simulink model "ZEH_PV_grid"  (R2020a)
settings: Solver=VariableStepAuto  StartTime=0.0  StopTime=24*60*60  RelTol=1e-3
InitFcn:
  | SENSE2_dat
values from neighbouring files (symbols this model uses):
  apv = [72 76 288 252 0 0 40 360 460 168 84]  *1E2    [ZEH_dat_summer.m]    (also in ZEH_dat_winter.m)
  cab = [0.206 0.29 0.36 285 335 ... (first row only)    [ZEH_dat_summer.m]    (also in ZEH_dat_winter.m)
  cons = [0.64,0.60,0.58,0.56,0.56,0.58,0.64,0.76,0.87,0.95,0.99,1.00,0.99,1.00,1.00,0.97,0.96,0.96,0.93,0.92,0.92,0.93,0.87,0.72]    [ZEH_dat_summer.m]    (also in ZEH_dat_winter.m = [0.67,0.63,0.60,0.59,0.59,0.60,0.74,0.86,0.85,0.96,0.96,0.95)
  inic = 0.00095    [ZEH_dat_summer.m]    (also in ZEH_dat_winter.m)
  irr = [0,0,0,0,0,0,0,0,0,0,0,0,0,0,0,0,0,0,0,0,0,0,0,0,0,0,0,0,0,0,0,0,0,0,0,0,0,0,0,0,0,0,0,0,0,0,0,0,0,0,0,0,0,0,0,0,0,0,0,0,0,0,0,0,0,0,0,0,0,0,0,0,0,0,0,0,0,0,0,0,0,0,0,0,0,0,0,0,0,0,0,0,0,0,0,0,0,0,0,0,0,0,0,0,0,0,0,0,0,0,0,0,0,0,0,0,0,0,0,0,0,0,0,0,0,0,0,0,0,0,0,0,0,0,0,0,0,0,0,0,0,0,0,0,0,0,0,0,0,0,0,0,0,0,0,0,0,0,0,0,0,0,0,0,0,0,0,0,0,0,0,0,0,0,0,0,0,0,0,0,0,0,0,0,0,0,0,0,0,0,0,0,0,0,0,0,0,0,0,0 ...(+12851 chars)    [ZEH_dat_summer.m]    (also in ZEH_dat_winter.m = zeros(1,length(irr)))
  lp = 0.002    [ZEH_dat_summer.m]    (also in ZEH_dat_winter.m)
  SL = [7.57 8.06 30.73 53.01 133.26 219.22 4.00 37.53 48.38 17.80 9.04]*1E-3    [ZEH_dat_summer.m]    (also in ZEH_dat_winter.m)
  time = [1,1.01666666666667,1.03333333333333,1.05000000000000,1.06666666666667,1.08333333333333,1.10000000000000,1.11666666666667,1.13333333333333,1.15000000000000,1.16666666666667,1.18333333333333,1.20000000000000,1.21666666666667,1.23333333333333,1.25000000000000,1.26666666666667,1.28333333333333,1.30000000000000,1.31666666666667,1.33333333333333,1.35000000000000,1.36666666666667,1.38333333333333,1.4000 ...(+22733 chars)    [ZEH_dat_summer.m]    (also in ZEH_dat_winter.m)
  to = 0.1    [ZEH_dat_summer.m]    (also in ZEH_dat_winter.m)
undefined symbols (not defined in the file or in its folder): A, B, C, D1, Dd, Delta, j
libraries: powerlib x166, simulink_extras x12, powerlib_meascontrol x11, simulink x2, factslib x2
(part 3 of 5)

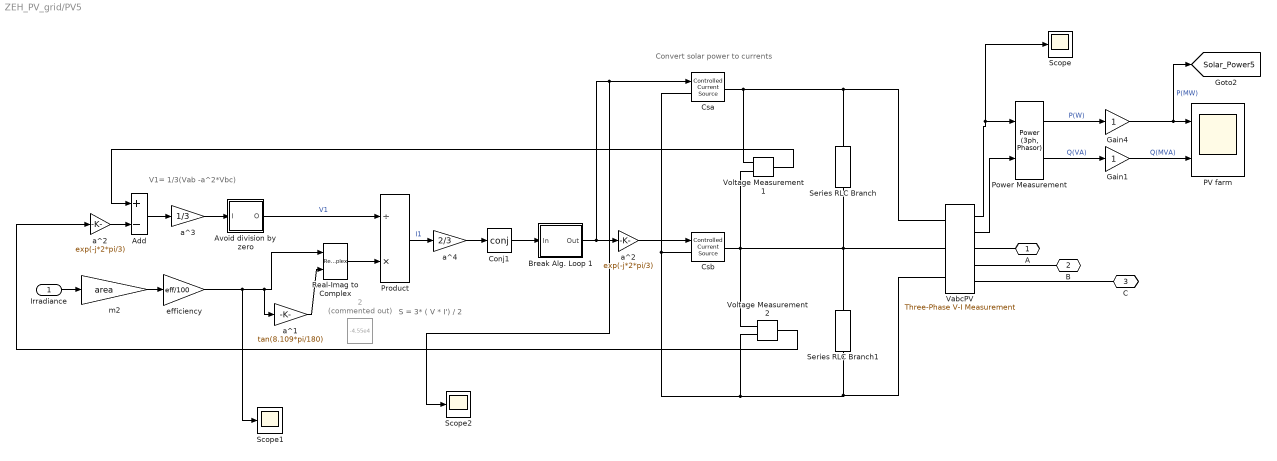
== system ZEH_PV_grid/PV5 ==
  note: Convert solar power to currents
  note: V1= 1/3(Vab -a^2*Vbc)
  note: S = 3* ( V * I') / 2
  Irradiance : Inport
  2 : Constant  Commented=on  Value=-4.55e4
  Add : Sum  Inputs=+-
  Avoid division by zero : Subsystem
  Break Alg. Loop 1 : Subsystem
  Conj1 : Math  Operator=conj  SignedPower=on  SaturateOnIntegerOverflow=on
  Csa : powerlib/Electrical Sources/Controlled Current Source  Initialize=on  Source_Type=AC  Amplitude=0  Phase=0  Frequency=50  Measurements=None
  Csb : powerlib/Electrical Sources/Controlled Current Source  Initialize=on  Source_Type=AC  Amplitude=0  Phase=0  Frequency=50  Measurements=None
  Gain1 : Gain
  Gain4 : Gain
  PV farm : Scope  NumInputPorts=2
  Power Measurement : powerlib_meascontrol/Measurements/Power (3ph, Phasor)
      settings: SourceProductBaseCode=PS
  Product : Product  Inputs=/*  InputSameDT=on  SaturateOnIntegerOverflow=on  OutDataTypeStr=Inherit: Same as first input
  Real-Imag to Complex : RealImagToComplex
  Scope : Scope
  Scope1 : Scope
  Scope2 : Scope
  Series RLC Branch : powerlib/Elements/Series RLC Branch  LConnTagsString=__new0  RConnTagsString=__new0  BranchType=R  Resistance=1e6  Inductance=1e-3  SetiL0=off  InitialCurrent=0  Capacitance=1e-6  Setx0=off  InitialVoltage=0  Measurements=None
  Series RLC Branch1 : powerlib/Elements/Series RLC Branch  LConnTagsString=__new0  RConnTagsString=__new0  BranchType=R  Resistance=1e6  Inductance=1e-3  SetiL0=off  InitialCurrent=0  Capacitance=1e-6  Setx0=off  InitialVoltage=0  Measurements=None
  VabcPV : powerlib/Measurements/Three-Phase V-I Measurement  VoltageMeasurement=phase-to-phase  SetLabelV=off  LabelV=V_Solar  Vpu=off  VpuLL=off  CurrentMeasurement=yes  SetLabelI=off  LabelI=I_Solar  Ipu=off  Pbase=2*1.5e6/0.9  Vbase=25e3  OutputType=Magnitude  PhasorSimulation=on  PSBequivalent=0
  Voltage Measurement1 : powerlib/Measurements/Voltage Measurement  PhasorSimulation=on  OutputType=Complex  PSBequivalent=0
  Voltage Measurement2 : powerlib/Measurements/Voltage Measurement  PhasorSimulation=on  OutputType=Complex  PSBequivalent=0
  a^1 : Gain  Gain=tan(8.109*pi/180)  SaturateOnIntegerOverflow=on  OutDataTypeStr=Inherit: Same as input  ParamDataTypeStr=Inherit: Same as input
  a^2 : Gain  Gain=exp(-j*2*pi/3)  SaturateOnIntegerOverflow=on  OutDataTypeStr=Inherit: Same as input  ParamDataTypeStr=Inherit: Same as input
  "a^2 " : Gain  Gain=exp(-j*2*pi/3)  SaturateOnIntegerOverflow=on  OutDataTypeStr=Inherit: Same as input  ParamDataTypeStr=Inherit: Same as input
  a^3 : Gain  Gain=1/3  SaturateOnIntegerOverflow=on  OutDataTypeStr=Inherit: Same as input  ParamDataTypeStr=Inherit: Same as input
  a^4 : Gain  Gain=2/3  SaturateOnIntegerOverflow=on  OutDataTypeStr=Inherit: Same as input  ParamDataTypeStr=Inherit: Same as input
  efficiency : Gain  Gain=eff/100
  m2 : Gain  Gain=area
  A : PMIOPort  Side=Right
  B : PMIOPort  Port=2  Side=Right
  C : PMIOPort  Port=3  Side=Right
  tag scope: Solar_Power5=global
  wires:
  VabcPV/1 -> Scope/1, Power Measurement/1
  Power Measurement/1 -> Gain4/1  "P(W)"
  VabcPV/2 -> Power Measurement/2
  Power Measurement/2 -> Gain1/1  "Q(VA)"
  Gain4/1 -> [Solar_Power5], PV farm/1  "P(MW)"
  Gain1/1 -> PV farm/2  "Q(MVA)"
  Product/1 -> a^4/1  "I1"
  efficiency/1 -> Scope1/1, a^1/1, Real-Imag to Complex/1
  Voltage Measurement2/1 -> "a^2 "/1
  a^4/1 -> Conj1/1
  Irradiance/1 -> m2/1
  Break Alg. Loop 1/1(Out) -> Scope2/1, Csa/1, a^2/1
  "a^2 "/1 -> Add/2
  Avoid division by zero/1(O) -> Product/1  "V1"
  a^2/1 -> Csb/1
  Conj1/1 -> Break Alg. Loop 1/1(In)
  a^1/1 -> Real-Imag to Complex/2
  m2/1 -> efficiency/1
  Add/1 -> a^3/1
  Voltage Measurement1/1 -> Add/1
  Real-Imag to Complex/1 -> Product/2
  a^3/1 -> Avoid division by zero/1(I)
  connections:
  B/RConn1 -- VabcPV/RConn2
  A/RConn1 -- VabcPV/RConn1
  VabcPV/RConn3 -- C/RConn1
  Series RLC Branch1/LConn1 -- Series RLC Branch/RConn1 -- VabcPV/LConn2 -- Voltage Measurement1/LConn2 -- Voltage Measurement2/LConn1 -- Csb/RConn1
  Series RLC Branch/LConn1 -- VabcPV/LConn1 -- Voltage Measurement1/LConn1 -- Csa/RConn1
  Series RLC Branch1/RConn1 -- VabcPV/LConn3 -- Voltage Measurement2/LConn2 -- Csa/LConn1 -- Csb/LConn1

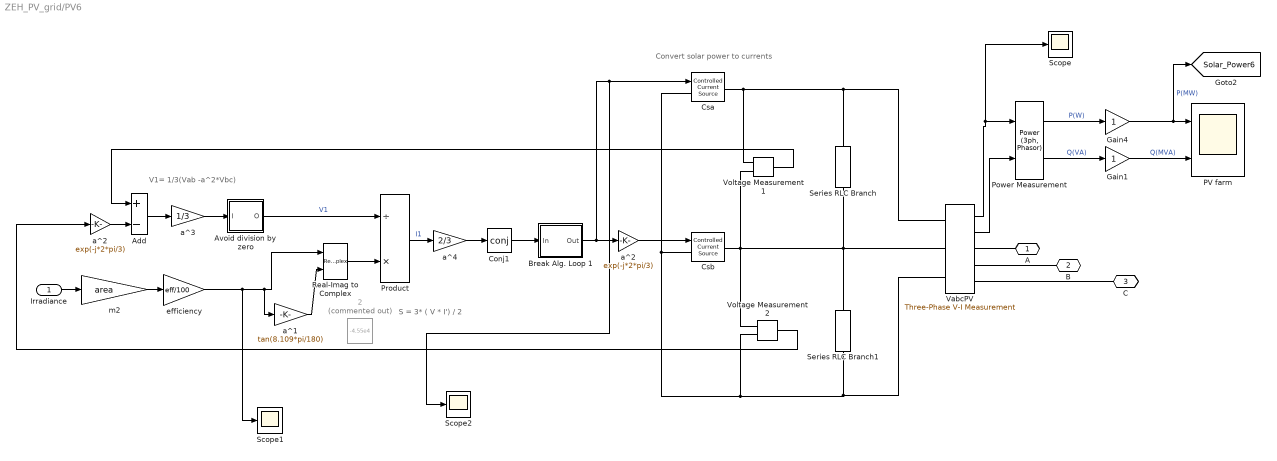
== system ZEH_PV_grid/PV6 ==
  note: S = 3* ( V * I') / 2
  note: V1= 1/3(Vab -a^2*Vbc)
  note: Convert solar power to currents
  Irradiance : Inport
  2 : Constant  Commented=on  Value=-4.55e4
  Add : Sum  Inputs=+-
  Avoid division by zero : Subsystem
  Break Alg. Loop 1 : Subsystem
  Conj1 : Math  Operator=conj  SignedPower=on  SaturateOnIntegerOverflow=on
  Csa : powerlib/Electrical Sources/Controlled Current Source  Initialize=on  Source_Type=AC  Amplitude=0  Phase=0  Frequency=50  Measurements=None
  Csb : powerlib/Electrical Sources/Controlled Current Source  Initialize=on  Source_Type=AC  Amplitude=0  Phase=0  Frequency=50  Measurements=None
  Gain1 : Gain
  Gain4 : Gain
  PV farm : Scope  NumInputPorts=2
  Power Measurement : powerlib_meascontrol/Measurements/Power (3ph, Phasor)
      settings: SourceProductBaseCode=PS
  Product : Product  Inputs=/*  InputSameDT=on  SaturateOnIntegerOverflow=on  OutDataTypeStr=Inherit: Same as first input
  Real-Imag to Complex : RealImagToComplex
  Scope : Scope
  Scope1 : Scope
  Scope2 : Scope
  Series RLC Branch : powerlib/Elements/Series RLC Branch  LConnTagsString=__new0  RConnTagsString=__new0  BranchType=R  Resistance=1e6  Inductance=1e-3  SetiL0=off  InitialCurrent=0  Capacitance=1e-6  Setx0=off  InitialVoltage=0  Measurements=None
  Series RLC Branch1 : powerlib/Elements/Series RLC Branch  LConnTagsString=__new0  RConnTagsString=__new0  BranchType=R  Resistance=1e6  Inductance=1e-3  SetiL0=off  InitialCurrent=0  Capacitance=1e-6  Setx0=off  InitialVoltage=0  Measurements=None
  VabcPV : powerlib/Measurements/Three-Phase V-I Measurement  VoltageMeasurement=phase-to-phase  SetLabelV=off  LabelV=V_Solar  Vpu=off  VpuLL=off  CurrentMeasurement=yes  SetLabelI=off  LabelI=I_Solar  Ipu=off  Pbase=2*1.5e6/0.9  Vbase=25e3  OutputType=Magnitude  PhasorSimulation=on  PSBequivalent=0
  Voltage Measurement1 : powerlib/Measurements/Voltage Measurement  PhasorSimulation=on  OutputType=Complex  PSBequivalent=0
  Voltage Measurement2 : powerlib/Measurements/Voltage Measurement  PhasorSimulation=on  OutputType=Complex  PSBequivalent=0
  a^1 : Gain  Gain=tan(8.109*pi/180)  SaturateOnIntegerOverflow=on  OutDataTypeStr=Inherit: Same as input  ParamDataTypeStr=Inherit: Same as input
  a^2 : Gain  Gain=exp(-j*2*pi/3)  SaturateOnIntegerOverflow=on  OutDataTypeStr=Inherit: Same as input  ParamDataTypeStr=Inherit: Same as input
  "a^2 " : Gain  Gain=exp(-j*2*pi/3)  SaturateOnIntegerOverflow=on  OutDataTypeStr=Inherit: Same as input  ParamDataTypeStr=Inherit: Same as input
  a^3 : Gain  Gain=1/3  SaturateOnIntegerOverflow=on  OutDataTypeStr=Inherit: Same as input  ParamDataTypeStr=Inherit: Same as input
  a^4 : Gain  Gain=2/3  SaturateOnIntegerOverflow=on  OutDataTypeStr=Inherit: Same as input  ParamDataTypeStr=Inherit: Same as input
  efficiency : Gain  Gain=eff/100
  m2 : Gain  Gain=area
  A : PMIOPort  Side=Right
  B : PMIOPort  Port=2  Side=Right
  C : PMIOPort  Port=3  Side=Right
  tag scope: Solar_Power6=global
  wires:
  a^3/1 -> Avoid division by zero/1(I)
  Real-Imag to Complex/1 -> Product/2
  Voltage Measurement1/1 -> Add/1
  Add/1 -> a^3/1
  m2/1 -> efficiency/1
  a^1/1 -> Real-Imag to Complex/2
  Conj1/1 -> Break Alg. Loop 1/1(In)
  a^2/1 -> Csb/1
  Avoid division by zero/1(O) -> Product/1  "V1"
  "a^2 "/1 -> Add/2
  Break Alg. Loop 1/1(Out) -> a^2/1, Csa/1, Scope2/1
  Irradiance/1 -> m2/1
  a^4/1 -> Conj1/1
  Voltage Measurement2/1 -> "a^2 "/1
  efficiency/1 -> Real-Imag to Complex/1, a^1/1, Scope1/1
  Product/1 -> a^4/1  "I1"
  Gain1/1 -> PV farm/2  "Q(MVA)"
  Gain4/1 -> PV farm/1, [Solar_Power6]  "P(MW)"
  Power Measurement/2 -> Gain1/1  "Q(VA)"
  VabcPV/2 -> Power Measurement/2
  Power Measurement/1 -> Gain4/1  "P(W)"
  VabcPV/1 -> Power Measurement/1, Scope/1
  connections:
  Csb/LConn1 -- Csa/LConn1 -- Voltage Measurement2/LConn2 -- VabcPV/LConn3 -- Series RLC Branch1/RConn1
  Csa/RConn1 -- Voltage Measurement1/LConn1 -- VabcPV/LConn1 -- Series RLC Branch/LConn1
  Csb/RConn1 -- Voltage Measurement2/LConn1 -- Voltage Measurement1/LConn2 -- VabcPV/LConn2 -- Series RLC Branch/RConn1 -- Series RLC Branch1/LConn1
  VabcPV/RConn3 -- C/RConn1
  A/RConn1 -- VabcPV/RConn1
  B/RConn1 -- VabcPV/RConn2

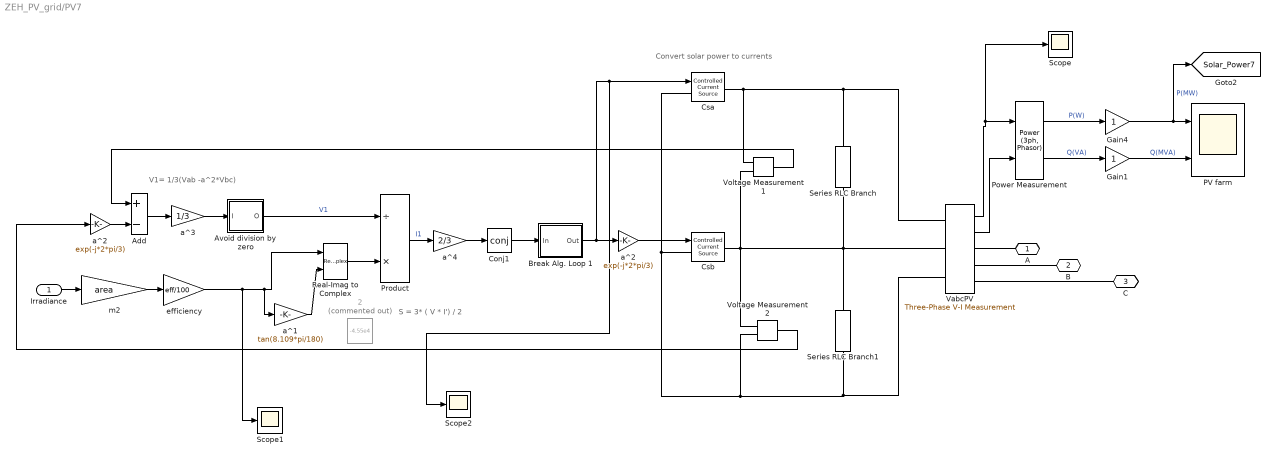
== system ZEH_PV_grid/PV7 ==
  note: Convert solar power to currents
  note: V1= 1/3(Vab -a^2*Vbc)
  note: S = 3* ( V * I') / 2
  Irradiance : Inport
  2 : Constant  Commented=on  Value=-4.55e4
  Add : Sum  Inputs=+-
  Avoid division by zero : Subsystem
  Break Alg. Loop 1 : Subsystem
  Conj1 : Math  Operator=conj  SignedPower=on  SaturateOnIntegerOverflow=on
  Csa : powerlib/Electrical Sources/Controlled Current Source  Initialize=on  Source_Type=AC  Amplitude=0  Phase=0  Frequency=50  Measurements=None
  Csb : powerlib/Electrical Sources/Controlled Current Source  Initialize=on  Source_Type=AC  Amplitude=0  Phase=0  Frequency=50  Measurements=None
  Gain1 : Gain
  Gain4 : Gain
  PV farm : Scope  NumInputPorts=2
  Power Measurement : powerlib_meascontrol/Measurements/Power (3ph, Phasor)
      settings: SourceProductBaseCode=PS
  Product : Product  Inputs=/*  InputSameDT=on  SaturateOnIntegerOverflow=on  OutDataTypeStr=Inherit: Same as first input
  Real-Imag to Complex : RealImagToComplex
  Scope : Scope
  Scope1 : Scope
  Scope2 : Scope
  Series RLC Branch : powerlib/Elements/Series RLC Branch  LConnTagsString=__new0  RConnTagsString=__new0  BranchType=R  Resistance=1e6  Inductance=1e-3  SetiL0=off  InitialCurrent=0  Capacitance=1e-6  Setx0=off  InitialVoltage=0  Measurements=None
  Series RLC Branch1 : powerlib/Elements/Series RLC Branch  LConnTagsString=__new0  RConnTagsString=__new0  BranchType=R  Resistance=1e6  Inductance=1e-3  SetiL0=off  InitialCurrent=0  Capacitance=1e-6  Setx0=off  InitialVoltage=0  Measurements=None
  VabcPV : powerlib/Measurements/Three-Phase V-I Measurement  VoltageMeasurement=phase-to-phase  SetLabelV=off  LabelV=V_Solar  Vpu=off  VpuLL=off  CurrentMeasurement=yes  SetLabelI=off  LabelI=I_Solar  Ipu=off  Pbase=2*1.5e6/0.9  Vbase=25e3  OutputType=Magnitude  PhasorSimulation=on  PSBequivalent=0
  Voltage Measurement1 : powerlib/Measurements/Voltage Measurement  PhasorSimulation=on  OutputType=Complex  PSBequivalent=0
  Voltage Measurement2 : powerlib/Measurements/Voltage Measurement  PhasorSimulation=on  OutputType=Complex  PSBequivalent=0
  a^1 : Gain  Gain=tan(8.109*pi/180)  SaturateOnIntegerOverflow=on  OutDataTypeStr=Inherit: Same as input  ParamDataTypeStr=Inherit: Same as input
  a^2 : Gain  Gain=exp(-j*2*pi/3)  SaturateOnIntegerOverflow=on  OutDataTypeStr=Inherit: Same as input  ParamDataTypeStr=Inherit: Same as input
  "a^2 " : Gain  Gain=exp(-j*2*pi/3)  SaturateOnIntegerOverflow=on  OutDataTypeStr=Inherit: Same as input  ParamDataTypeStr=Inherit: Same as input
  a^3 : Gain  Gain=1/3  SaturateOnIntegerOverflow=on  OutDataTypeStr=Inherit: Same as input  ParamDataTypeStr=Inherit: Same as input
  a^4 : Gain  Gain=2/3  SaturateOnIntegerOverflow=on  OutDataTypeStr=Inherit: Same as input  ParamDataTypeStr=Inherit: Same as input
  efficiency : Gain  Gain=eff/100
  m2 : Gain  Gain=area
  A : PMIOPort  Side=Right
  B : PMIOPort  Port=2  Side=Right
  C : PMIOPort  Port=3  Side=Right
  tag scope: Solar_Power7=global
  wires:
  VabcPV/1 -> Scope/1, Power Measurement/1
  Power Measurement/1 -> Gain4/1  "P(W)"
  VabcPV/2 -> Power Measurement/2
  Power Measurement/2 -> Gain1/1  "Q(VA)"
  Gain4/1 -> [Solar_Power7], PV farm/1  "P(MW)"
  Gain1/1 -> PV farm/2  "Q(MVA)"
  Product/1 -> a^4/1  "I1"
  efficiency/1 -> Scope1/1, a^1/1, Real-Imag to Complex/1
  Voltage Measurement2/1 -> "a^2 "/1
  a^4/1 -> Conj1/1
  Irradiance/1 -> m2/1
  Break Alg. Loop 1/1(Out) -> Scope2/1, Csa/1, a^2/1
  "a^2 "/1 -> Add/2
  Avoid division by zero/1(O) -> Product/1  "V1"
  a^2/1 -> Csb/1
  Conj1/1 -> Break Alg. Loop 1/1(In)
  a^1/1 -> Real-Imag to Complex/2
  m2/1 -> efficiency/1
  Add/1 -> a^3/1
  Voltage Measurement1/1 -> Add/1
  Real-Imag to Complex/1 -> Product/2
  a^3/1 -> Avoid division by zero/1(I)
  connections:
  B/RConn1 -- VabcPV/RConn2
  A/RConn1 -- VabcPV/RConn1
  VabcPV/RConn3 -- C/RConn1
  Series RLC Branch1/LConn1 -- Series RLC Branch/RConn1 -- VabcPV/LConn2 -- Voltage Measurement1/LConn2 -- Voltage Measurement2/LConn1 -- Csb/RConn1
  Series RLC Branch/LConn1 -- VabcPV/LConn1 -- Voltage Measurement1/LConn1 -- Csa/RConn1
  Series RLC Branch1/RConn1 -- VabcPV/LConn3 -- Voltage Measurement2/LConn2 -- Csa/LConn1 -- Csb/LConn1

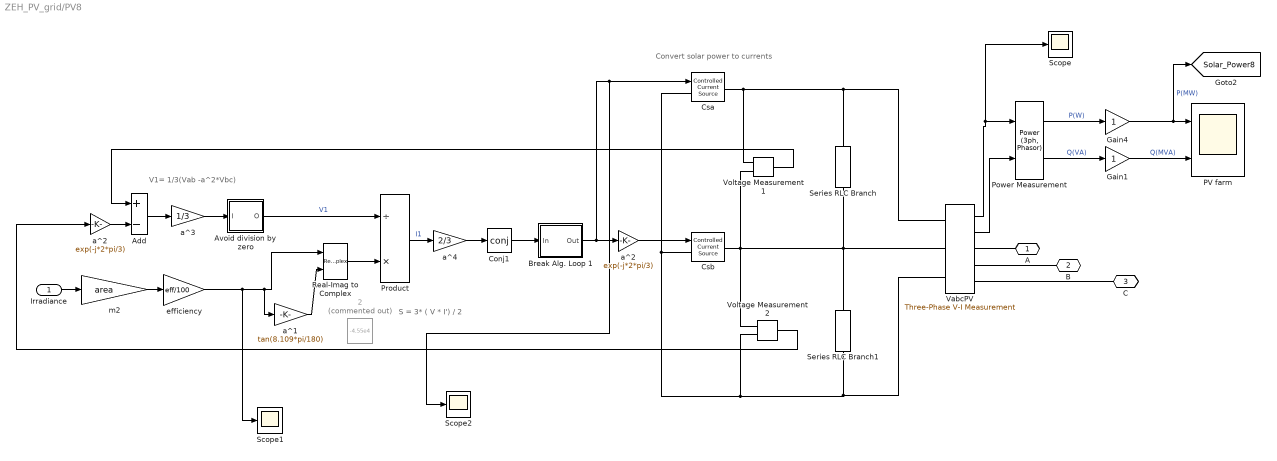
== system ZEH_PV_grid/PV8 ==
  note: S = 3* ( V * I') / 2
  note: V1= 1/3(Vab -a^2*Vbc)
  note: Convert solar power to currents
  Irradiance : Inport
  2 : Constant  Commented=on  Value=-4.55e4
  Add : Sum  Inputs=+-
  Avoid division by zero : Subsystem
  Break Alg. Loop 1 : Subsystem
  Conj1 : Math  Operator=conj  SignedPower=on  SaturateOnIntegerOverflow=on
  Csa : powerlib/Electrical Sources/Controlled Current Source  Initialize=on  Source_Type=AC  Amplitude=0  Phase=0  Frequency=50  Measurements=None
  Csb : powerlib/Electrical Sources/Controlled Current Source  Initialize=on  Source_Type=AC  Amplitude=0  Phase=0  Frequency=50  Measurements=None
  Gain1 : Gain
  Gain4 : Gain
  PV farm : Scope  NumInputPorts=2
  Power Measurement : powerlib_meascontrol/Measurements/Power (3ph, Phasor)
      settings: SourceProductBaseCode=PS
  Product : Product  Inputs=/*  InputSameDT=on  SaturateOnIntegerOverflow=on  OutDataTypeStr=Inherit: Same as first input
  Real-Imag to Complex : RealImagToComplex
  Scope : Scope
  Scope1 : Scope
  Scope2 : Scope
  Series RLC Branch : powerlib/Elements/Series RLC Branch  LConnTagsString=__new0  RConnTagsString=__new0  BranchType=R  Resistance=1e6  Inductance=1e-3  SetiL0=off  InitialCurrent=0  Capacitance=1e-6  Setx0=off  InitialVoltage=0  Measurements=None
  Series RLC Branch1 : powerlib/Elements/Series RLC Branch  LConnTagsString=__new0  RConnTagsString=__new0  BranchType=R  Resistance=1e6  Inductance=1e-3  SetiL0=off  InitialCurrent=0  Capacitance=1e-6  Setx0=off  InitialVoltage=0  Measurements=None
  VabcPV : powerlib/Measurements/Three-Phase V-I Measurement  VoltageMeasurement=phase-to-phase  SetLabelV=off  LabelV=V_Solar  Vpu=off  VpuLL=off  CurrentMeasurement=yes  SetLabelI=off  LabelI=I_Solar  Ipu=off  Pbase=2*1.5e6/0.9  Vbase=25e3  OutputType=Magnitude  PhasorSimulation=on  PSBequivalent=0
  Voltage Measurement1 : powerlib/Measurements/Voltage Measurement  PhasorSimulation=on  OutputType=Complex  PSBequivalent=0
  Voltage Measurement2 : powerlib/Measurements/Voltage Measurement  PhasorSimulation=on  OutputType=Complex  PSBequivalent=0
  a^1 : Gain  Gain=tan(8.109*pi/180)  SaturateOnIntegerOverflow=on  OutDataTypeStr=Inherit: Same as input  ParamDataTypeStr=Inherit: Same as input
  a^2 : Gain  Gain=exp(-j*2*pi/3)  SaturateOnIntegerOverflow=on  OutDataTypeStr=Inherit: Same as input  ParamDataTypeStr=Inherit: Same as input
  "a^2 " : Gain  Gain=exp(-j*2*pi/3)  SaturateOnIntegerOverflow=on  OutDataTypeStr=Inherit: Same as input  ParamDataTypeStr=Inherit: Same as input
  a^3 : Gain  Gain=1/3  SaturateOnIntegerOverflow=on  OutDataTypeStr=Inherit: Same as input  ParamDataTypeStr=Inherit: Same as input
  a^4 : Gain  Gain=2/3  SaturateOnIntegerOverflow=on  OutDataTypeStr=Inherit: Same as input  ParamDataTypeStr=Inherit: Same as input
  efficiency : Gain  Gain=eff/100
  m2 : Gain  Gain=area
  A : PMIOPort  Side=Right
  B : PMIOPort  Port=2  Side=Right
  C : PMIOPort  Port=3  Side=Right
  tag scope: Solar_Power8=global
  wires:
  a^3/1 -> Avoid division by zero/1(I)
  Real-Imag to Complex/1 -> Product/2
  Voltage Measurement1/1 -> Add/1
  Add/1 -> a^3/1
  m2/1 -> efficiency/1
  a^1/1 -> Real-Imag to Complex/2
  Conj1/1 -> Break Alg. Loop 1/1(In)
  a^2/1 -> Csb/1
  Avoid division by zero/1(O) -> Product/1  "V1"
  "a^2 "/1 -> Add/2
  Break Alg. Loop 1/1(Out) -> a^2/1, Csa/1, Scope2/1
  Irradiance/1 -> m2/1
  a^4/1 -> Conj1/1
  Voltage Measurement2/1 -> "a^2 "/1
  efficiency/1 -> Real-Imag to Complex/1, a^1/1, Scope1/1
  Product/1 -> a^4/1  "I1"
  Gain1/1 -> PV farm/2  "Q(MVA)"
  Gain4/1 -> PV farm/1, [Solar_Power8]  "P(MW)"
  Power Measurement/2 -> Gain1/1  "Q(VA)"
  VabcPV/2 -> Power Measurement/2
  Power Measurement/1 -> Gain4/1  "P(W)"
  VabcPV/1 -> Power Measurement/1, Scope/1
  connections:
  Csb/LConn1 -- Csa/LConn1 -- Voltage Measurement2/LConn2 -- VabcPV/LConn3 -- Series RLC Branch1/RConn1
  Csa/RConn1 -- Voltage Measurement1/LConn1 -- VabcPV/LConn1 -- Series RLC Branch/LConn1
  Csb/RConn1 -- Voltage Measurement2/LConn1 -- Voltage Measurement1/LConn2 -- VabcPV/LConn2 -- Series RLC Branch/RConn1 -- Series RLC Branch1/LConn1
  VabcPV/RConn3 -- C/RConn1
  A/RConn1 -- VabcPV/RConn1
  B/RConn1 -- VabcPV/RConn2

== system ZEH_PV_grid/PV9 ==
  note: Convert solar power to currents
  note: V1= 1/3(Vab -a^2*Vbc)
  note: S = 3* ( V * I') / 2
  Irradiance : Inport
  2 : Constant  Commented=on  Value=-4.55e4
  Add : Sum  Inputs=+-
  Avoid division by zero : Subsystem
  Break Alg. Loop 1 : Subsystem
  Conj1 : Math  Operator=conj  SignedPower=on  SaturateOnIntegerOverflow=on
  Csa : powerlib/Electrical Sources/Controlled Current Source  Initialize=on  Source_Type=AC  Amplitude=0  Phase=0  Frequency=50  Measurements=None
  Csb : powerlib/Electrical Sources/Controlled Current Source  Initialize=on  Source_Type=AC  Amplitude=0  Phase=0  Frequency=50  Measurements=None
  Gain1 : Gain
  Gain4 : Gain
  PV farm : Scope  NumInputPorts=2
  Power Measurement : powerlib_meascontrol/Measurements/Power (3ph, Phasor)
      settings: SourceProductBaseCode=PS
  Product : Product  Inputs=/*  InputSameDT=on  SaturateOnIntegerOverflow=on  OutDataTypeStr=Inherit: Same as first input
  Real-Imag to Complex : RealImagToComplex
  Scope : Scope
  Scope1 : Scope
  Scope2 : Scope
  Series RLC Branch : powerlib/Elements/Series RLC Branch  LConnTagsString=__new0  RConnTagsString=__new0  BranchType=R  Resistance=1e6  Inductance=1e-3  SetiL0=off  InitialCurrent=0  Capacitance=1e-6  Setx0=off  InitialVoltage=0  Measurements=None
  Series RLC Branch1 : powerlib/Elements/Series RLC Branch  LConnTagsString=__new0  RConnTagsString=__new0  BranchType=R  Resistance=1e6  Inductance=1e-3  SetiL0=off  InitialCurrent=0  Capacitance=1e-6  Setx0=off  InitialVoltage=0  Measurements=None
  VabcPV : powerlib/Measurements/Three-Phase V-I Measurement  VoltageMeasurement=phase-to-phase  SetLabelV=off  LabelV=V_Solar  Vpu=off  VpuLL=off  CurrentMeasurement=yes  SetLabelI=off  LabelI=I_Solar  Ipu=off  Pbase=2*1.5e6/0.9  Vbase=25e3  OutputType=Magnitude  PhasorSimulation=on  PSBequivalent=0
  Voltage Measurement1 : powerlib/Measurements/Voltage Measurement  PhasorSimulation=on  OutputType=Complex  PSBequivalent=0
  Voltage Measurement2 : powerlib/Measurements/Voltage Measurement  PhasorSimulation=on  OutputType=Complex  PSBequivalent=0
  a^1 : Gain  Gain=tan(8.109*pi/180)  SaturateOnIntegerOverflow=on  OutDataTypeStr=Inherit: Same as input  ParamDataTypeStr=Inherit: Same as input
  a^2 : Gain  Gain=exp(-j*2*pi/3)  SaturateOnIntegerOverflow=on  OutDataTypeStr=Inherit: Same as input  ParamDataTypeStr=Inherit: Same as input
  "a^2 " : Gain  Gain=exp(-j*2*pi/3)  SaturateOnIntegerOverflow=on  OutDataTypeStr=Inherit: Same as input  ParamDataTypeStr=Inherit: Same as input
  a^3 : Gain  Gain=1/3  SaturateOnIntegerOverflow=on  OutDataTypeStr=Inherit: Same as input  ParamDataTypeStr=Inherit: Same as input
  a^4 : Gain  Gain=2/3  SaturateOnIntegerOverflow=on  OutDataTypeStr=Inherit: Same as input  ParamDataTypeStr=Inherit: Same as input
  efficiency : Gain  Gain=eff/100
  m2 : Gain  Gain=area
  A : PMIOPort  Side=Right
  B : PMIOPort  Port=2  Side=Right
  C : PMIOPort  Port=3  Side=Right
  tag scope: Solar_Power9=global
  wires:
  VabcPV/1 -> Scope/1, Power Measurement/1
  Power Measurement/1 -> Gain4/1  "P(W)"
  VabcPV/2 -> Power Measurement/2
  Power Measurement/2 -> Gain1/1  "Q(VA)"
  Gain4/1 -> [Solar_Power9], PV farm/1  "P(MW)"
  Gain1/1 -> PV farm/2  "Q(MVA)"
  Product/1 -> a^4/1  "I1"
  efficiency/1 -> Scope1/1, a^1/1, Real-Imag to Complex/1
  Voltage Measurement2/1 -> "a^2 "/1
  a^4/1 -> Conj1/1
  Irradiance/1 -> m2/1
  Break Alg. Loop 1/1(Out) -> Scope2/1, Csa/1, a^2/1
  "a^2 "/1 -> Add/2
  Avoid division by zero/1(O) -> Product/1  "V1"
  a^2/1 -> Csb/1
  Conj1/1 -> Break Alg. Loop 1/1(In)
  a^1/1 -> Real-Imag to Complex/2
  m2/1 -> efficiency/1
  Add/1 -> a^3/1
  Voltage Measurement1/1 -> Add/1
  Real-Imag to Complex/1 -> Product/2
  a^3/1 -> Avoid division by zero/1(I)
  connections:
  B/RConn1 -- VabcPV/RConn2
  A/RConn1 -- VabcPV/RConn1
  VabcPV/RConn3 -- C/RConn1
  Series RLC Branch1/LConn1 -- Series RLC Branch/RConn1 -- VabcPV/LConn2 -- Voltage Measurement1/LConn2 -- Voltage Measurement2/LConn1 -- Csb/RConn1
  Series RLC Branch/LConn1 -- VabcPV/LConn1 -- Voltage Measurement1/LConn1 -- Csa/RConn1
  Series RLC Branch1/RConn1 -- VabcPV/LConn3 -- Voltage Measurement2/LConn2 -- Csa/LConn1 -- Csb/LConn1

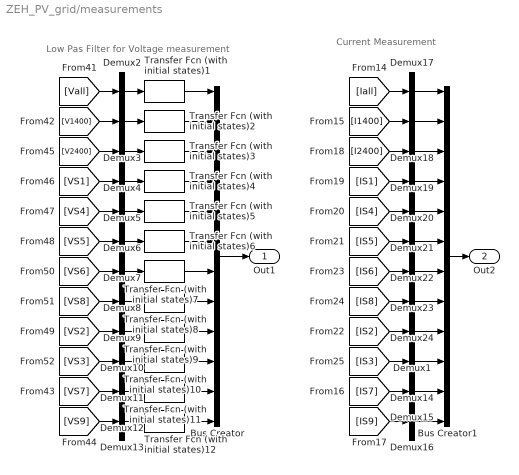
== system ZEH_PV_grid/measurements ==
  note: Current Measurement
  note: Low Pas Filter for Voltage measurement
  Bus Creator : BusCreator  Inputs=12
  Bus Creator1 : BusCreator  Inputs=12
  Demux{1..24} (24 alike) : Demux  Outputs=3
  Transfer Fcn (with initial states){1..12} (12 alike) : simulink_extras/Additional Linear/Transfer Fcn (with initial states)  N=[1]  D="[lp  1]"  X0=inic
  Out1 : Outport
  Out2 : Outport  Port=2
  wires:
  Bus Creator/1 -> Out1/1
  Transfer Fcn (with initial states)10/1 -> Bus Creator/10
  Transfer Fcn (with initial states)8/1 -> Bus Creator/8
  Transfer Fcn (with initial states)7/1 -> Bus Creator/7
  Transfer Fcn (with initial states)4/1 -> Bus Creator/4
  Transfer Fcn (with initial states)6/1 -> Bus Creator/6
  [V2400] -> Demux4/1
  Transfer Fcn (with initial states)1/1 -> Bus Creator/1
  [VS4] -> Demux6/1
  Demux12/2 -> Transfer Fcn (with initial states)11/1
  [VS6] -> Demux8/1
  Demux13/2 -> Transfer Fcn (with initial states)12/1
  Demux11/2 -> Transfer Fcn (with initial states)10/1
  Transfer Fcn (with initial states)5/1 -> Bus Creator/5
  Demux10/2 -> Transfer Fcn (with initial states)9/1
  Demux8/2 -> Transfer Fcn (with initial states)7/1
  [VS9] -> Demux13/1
  Demux7/2 -> Transfer Fcn (with initial states)6/1
  Demux9/2 -> Transfer Fcn (with initial states)8/1
  Demux2/2 -> Transfer Fcn (with initial states)1/1
  Demux6/2 -> Transfer Fcn (with initial states)5/1
  [VS5] -> Demux7/1
  [Vall] -> Demux2/1
  Demux4/2 -> Transfer Fcn (with initial states)3/1
  [V1400] -> Demux3/1
  [VS1] -> Demux5/1
  Demux5/2 -> Transfer Fcn (with initial states)4/1
  Transfer Fcn (with initial states)9/1 -> Bus Creator/9
  [VS2] -> Demux10/1
  [VS8] -> Demux9/1
  Transfer Fcn (with initial states)3/1 -> Bus Creator/3
  Transfer Fcn (with initial states)12/1 -> Bus Creator/12
  Demux3/2 -> Transfer Fcn (with initial states)2/1
  Transfer Fcn (with initial states)2/1 -> Bus Creator/2
  [VS3] -> Demux11/1
  [VS7] -> Demux12/1
  Transfer Fcn (with initial states)11/1 -> Bus Creator/11
  [IS7] -> Demux15/1
  [IS3] -> Demux14/1
  [IS8] -> Demux24/1
  [IS2] -> Demux1/1
  [IS1] -> Demux20/1
  [I1400] -> Demux18/1
  [Iall] -> Demux17/1
  [IS5] -> Demux22/1
  [IS9] -> Demux16/1
  [IS6] -> Demux23/1
  [IS4] -> Demux21/1
  [I2400] -> Demux19/1
  Demux16/2 -> Bus Creator1/12
  Demux20/2 -> Bus Creator1/4
  Demux19/2 -> Bus Creator1/3
  Demux15/2 -> Bus Creator1/11
  Bus Creator1/1 -> Out2/1
  Demux18/2 -> Bus Creator1/2
  Demux1/2 -> Bus Creator1/9
  Demux22/2 -> Bus Creator1/6
  Demux14/2 -> Bus Creator1/10
  Demux21/2 -> Bus Creator1/5
  Demux23/2 -> Bus Creator1/7
  Demux24/2 -> Bus Creator1/8
  Demux17/2 -> Bus Creator1/1

== system ZEH_PV_grid/ Irradiance curve/Irradiance ==
  1-D Lookup IRRADIANCE Table : Lookup_n-D  NumberOfTableDimensions=1  BreakpointsForDimension1=time  BeginIndexSearchUsingPreviousIndexResult=on  Table=irr  InternalRulePriority=Speed  RndMeth=Simplest  InputSameDT=on
  Add : Sum
  Clock1 : Clock
  Constant1 : Constant
  Second-->Hour : Gain  Gain=1/(60*60)
  " " : Outport  VectorParamsAs1DForOutWhenUnconnected=off
  wires:
  Constant1/1 -> Add/2
  Add/1 -> 1-D Lookup IRRADIANCE Table/1  "Hour of the day"
  1-D Lookup IRRADIANCE Table/1 -> " "/1
  Clock1/1 -> Second-->Hour/1
  Second-->Hour/1 -> Add/1

== system ZEH_PV_grid/ Irradiance curve/Partial Shading ==
  Add : Sum
  Clock : Clock
  Compare To Constant : simulink/Logic and Bit Operations/Compare To Constant  relop=>=  const=Ton  OutDataTypeStr=boolean
  Compare To Constant1 : simulink/Logic and Bit Operations/Compare To Constant  relop=<  const=Toff  OutDataTypeStr=boolean
  Constant : Constant  Value=Factor
  Logical Operator : Logic  AllPortsSameDT=off  OutDataTypeStr=float('double')
  Logical Operator1 : Logic  Operator=NOT  AllPortsSameDT=off  OutDataTypeStr=float('double')
  Product : Product
  Out : Outport  VectorParamsAs1DForOutWhenUnconnected=off
  wires:
  Add/1 -> Out/1
  Product/1 -> Add/2
  Constant/1 -> Product/2
  Compare To Constant/1 -> Logical Operator/1
  Clock/1 -> Compare To Constant1/1, Compare To Constant/1
  Compare To Constant1/1 -> Logical Operator/2
  Logical Operator/1 -> Logical Operator1/1, Product/1
  Logical Operator1/1 -> Add/1

== system ZEH_PV_grid/L1/Avoid division by zero ==
  I : Inport
  Complex to Magnitude-Angle : ComplexToMagnitudeAngle
  Magnitude-Angle to Complex : MagnitudeAngleToComplex
  Saturation1 : Saturate  UpperLimit=inf  LowerLimit=1e-6
  O : Outport  VectorParamsAs1DForOutWhenUnconnected=off
  wires:
  I/1 -> Complex to Magnitude-Angle/1
  Saturation1/1 -> Magnitude-Angle to Complex/1
  Complex to Magnitude-Angle/1 -> Saturation1/1
  Magnitude-Angle to Complex/1 -> O/1
  Complex to Magnitude-Angle/2 -> Magnitude-Angle to Complex/2

== system ZEH_PV_grid/L1/Break Alg. Loop 1 ==
  In : Inport
  Complex to Real-Imag : ComplexToRealImag
  Real-Imag to Complex : RealImagToComplex
  imag : Subsystem  mask(Transfer Function with Initial Outputs){N=[1], D=[to  1], Y0=0, U0=0}
      mask prompts: N "Numerator:"; D "Denominator:"; Y0 "Initial output:"; U0 "Initial input:"
      mask help: Vector expressions for numerator, and denominator. Coefficients are in descending powers of s.
      mask init:
      | [A,B,C,Dd]=tf2ss(N,D);if (isempty(Y0));[m,n]=size(A);X0=zeros(1,m); end; if (isempty(U0));[m,p]=size(B);U0=zeros(1,p);end;X0=getxo(A,B,C,Dd,U0,Y0,0);
      mask Help: Specify the initial output for the transfer function.  An optimization routine attempts to determine the appropriate initial states so that the specified initial output is achieved.  For more details, see the m-file getxo.m
      mask Display: dpoly(N,D,'s')
  real : Subsystem  mask(Transfer Function with Initial Outputs){N=[1], D=[to 1], Y0=0, U0=0}
      mask prompts: N "Numerator:"; D "Denominator:"; Y0 "Initial output:"; U0 "Initial input:"
      mask help: Vector expressions for numerator, and denominator. Coefficients are in descending powers of s.
      mask init:
      | [A,B,C,Dd]=tf2ss(N,D);if (isempty(Y0));[m,n]=size(A);X0=zeros(1,m); end; if (isempty(U0));[m,p]=size(B);U0=zeros(1,p);end;X0=getxo(A,B,C,Dd,U0,Y0,0);
      mask Help: Specify the initial output for the transfer function.  An optimization routine attempts to determine the appropriate initial states so that the specified initial output is achieved.  For more details, see the m-file getxo.m
      mask Display: dpoly(N,D,'s')
  Out : Outport  VectorParamsAs1DForOutWhenUnconnected=off
  wires:
  Complex to Real-Imag/1 -> real/1(In1)
  Complex to Real-Imag/2 -> imag/1(In1)
  In/1 -> Complex to Real-Imag/1
  Real-Imag to Complex/1 -> Out/1
  real/1(Out1) -> Real-Imag to Complex/1
  imag/1(Out1) -> Real-Imag to Complex/2

== system ZEH_PV_grid/L1/Load ==
  1 : Constant
  Add : Sum
  Clock : Clock
  Constant : Constant
  Constant1 : Constant  Value=15/24
  Divide : Product  Inputs=*/
  Manual Switch : ManualSwitch
  Mux : Mux  Inputs=2
  P nom : Constant  Value=-nomPower*1e6
  Power consumption : Lookup_n-D  NumberOfTableDimensions=1  BreakpointsForDimension1=[1:timestep/60:24]  BeginIndexSearchUsingPreviousIndexResult=on  Table=datas  InternalRulePriority=Speed  RndMeth=Simplest  InputSameDT=on
  Power factor : Constant  Value=PF^2
  Product : Product
  Product1 : Product
  Scope : Scope
  Second-->Hour : Gain  Gain=1/(60*60)
  Sqrt : Sqrt  SaturateOnIntegerOverflow=on
  Sum : Sum  Inputs=-+
  PQ : Outport  VectorParamsAs1DForOutWhenUnconnected=off
  wires:
  Constant/1 -> Add/2
  1/1 -> Sum/1, Divide/1
  Second-->Hour/1 -> Add/1
  Sum/1 -> Sqrt/1
  Power factor/1 -> Divide/2
  Add/1 -> Power consumption/1
  P nom/1 -> Product/2
  Clock/1 -> Second-->Hour/1
  Sqrt/1 -> Product1/2
  Product/1 -> Product1/1, Mux/1
  Divide/1 -> Sum/2
  Product1/1 -> Mux/2
  Power consumption/1 -> Manual Switch/1
  Manual Switch/1 -> Product/1
  Constant1/1 -> Manual Switch/2
  Mux/1 -> Scope/1, PQ/1

== system ZEH_PV_grid/L10/Avoid division by zero ==
  I : Inport
  Complex to Magnitude-Angle : ComplexToMagnitudeAngle
  Magnitude-Angle to Complex : MagnitudeAngleToComplex
  Saturation1 : Saturate  UpperLimit=inf  LowerLimit=1e-6
  O : Outport  VectorParamsAs1DForOutWhenUnconnected=off
  wires:
  Complex to Magnitude-Angle/2 -> Magnitude-Angle to Complex/2
  Magnitude-Angle to Complex/1 -> O/1
  Complex to Magnitude-Angle/1 -> Saturation1/1
  Saturation1/1 -> Magnitude-Angle to Complex/1
  I/1 -> Complex to Magnitude-Angle/1

== system ZEH_PV_grid/L10/Break Alg. Loop 1 ==
  In : Inport
  Complex to Real-Imag : ComplexToRealImag
  Real-Imag to Complex : RealImagToComplex
  imag : Subsystem  mask(Transfer Function with Initial Outputs){N=[1], D=[to  1], Y0=0, U0=0}
      mask prompts: N "Numerator:"; D "Denominator:"; Y0 "Initial output:"; U0 "Initial input:"
      mask help: Vector expressions for numerator, and denominator. Coefficients are in descending powers of s.
      mask init:
      | [A,B,C,Dd]=tf2ss(N,D);if (isempty(Y0));[m,n]=size(A);X0=zeros(1,m); end; if (isempty(U0));[m,p]=size(B);U0=zeros(1,p);end;X0=getxo(A,B,C,Dd,U0,Y0,0);
      mask Help: Specify the initial output for the transfer function.  An optimization routine attempts to determine the appropriate initial states so that the specified initial output is achieved.  For more details, see the m-file getxo.m
      mask Display: dpoly(N,D,'s')
  real : Subsystem  mask(Transfer Function with Initial Outputs){N=[1], D=[to 1], Y0=0, U0=0}
      mask prompts: N "Numerator:"; D "Denominator:"; Y0 "Initial output:"; U0 "Initial input:"
      mask help: Vector expressions for numerator, and denominator. Coefficients are in descending powers of s.
      mask init:
      | [A,B,C,Dd]=tf2ss(N,D);if (isempty(Y0));[m,n]=size(A);X0=zeros(1,m); end; if (isempty(U0));[m,p]=size(B);U0=zeros(1,p);end;X0=getxo(A,B,C,Dd,U0,Y0,0);
      mask Help: Specify the initial output for the transfer function.  An optimization routine attempts to determine the appropriate initial states so that the specified initial output is achieved.  For more details, see the m-file getxo.m
      mask Display: dpoly(N,D,'s')
  Out : Outport  VectorParamsAs1DForOutWhenUnconnected=off
  wires:
  imag/1(Out1) -> Real-Imag to Complex/2
  real/1(Out1) -> Real-Imag to Complex/1
  Real-Imag to Complex/1 -> Out/1
  In/1 -> Complex to Real-Imag/1
  Complex to Real-Imag/2 -> imag/1(In1)
  Complex to Real-Imag/1 -> real/1(In1)

== system ZEH_PV_grid/L10/Load ==
  1 : Constant
  Add : Sum
  Clock : Clock
  Constant : Constant
  Constant1 : Constant  Value=15/24
  Divide : Product  Inputs=*/
  Manual Switch : ManualSwitch
  Mux : Mux  Inputs=2
  P nom : Constant  Value=-nomPower*1e6
  Power consumption : Lookup_n-D  NumberOfTableDimensions=1  BreakpointsForDimension1=[1:timestep/60:24]  BeginIndexSearchUsingPreviousIndexResult=on  Table=datas  InternalRulePriority=Speed  RndMeth=Simplest  InputSameDT=on
  Power factor : Constant  Value=PF^2
  Product : Product
  Product1 : Product
  Scope : Scope
  Second-->Hour : Gain  Gain=1/(60*60)
  Sqrt : Sqrt  SaturateOnIntegerOverflow=on
  Sum : Sum  Inputs=-+
  PQ : Outport  VectorParamsAs1DForOutWhenUnconnected=off
  wires:
  Mux/1 -> PQ/1, Scope/1
  Constant1/1 -> Manual Switch/2
  Manual Switch/1 -> Product/1
  Power consumption/1 -> Manual Switch/1
  Product1/1 -> Mux/2
  Divide/1 -> Sum/2
  Product/1 -> Mux/1, Product1/1
  Sqrt/1 -> Product1/2
  Clock/1 -> Second-->Hour/1
  P nom/1 -> Product/2
  Add/1 -> Power consumption/1
  Power factor/1 -> Divide/2
  Sum/1 -> Sqrt/1
  Second-->Hour/1 -> Add/1
  1/1 -> Divide/1, Sum/1
  Constant/1 -> Add/2

== system ZEH_PV_grid/L11/Avoid division by zero ==
  I : Inport
  Complex to Magnitude-Angle : ComplexToMagnitudeAngle
  Magnitude-Angle to Complex : MagnitudeAngleToComplex
  Saturation1 : Saturate  UpperLimit=inf  LowerLimit=1e-6
  O : Outport  VectorParamsAs1DForOutWhenUnconnected=off
  wires:
  I/1 -> Complex to Magnitude-Angle/1
  Saturation1/1 -> Magnitude-Angle to Complex/1
  Complex to Magnitude-Angle/1 -> Saturation1/1
  Magnitude-Angle to Complex/1 -> O/1
  Complex to Magnitude-Angle/2 -> Magnitude-Angle to Complex/2

== system ZEH_PV_grid/L11/Break Alg. Loop 1 ==
  In : Inport
  Complex to Real-Imag : ComplexToRealImag
  Real-Imag to Complex : RealImagToComplex
  imag : Subsystem  mask(Transfer Function with Initial Outputs){N=[1], D=[to  1], Y0=0, U0=0}
      mask prompts: N "Numerator:"; D "Denominator:"; Y0 "Initial output:"; U0 "Initial input:"
      mask help: Vector expressions for numerator, and denominator. Coefficients are in descending powers of s.
      mask init:
      | [A,B,C,Dd]=tf2ss(N,D);if (isempty(Y0));[m,n]=size(A);X0=zeros(1,m); end; if (isempty(U0));[m,p]=size(B);U0=zeros(1,p);end;X0=getxo(A,B,C,Dd,U0,Y0,0);
      mask Help: Specify the initial output for the transfer function.  An optimization routine attempts to determine the appropriate initial states so that the specified initial output is achieved.  For more details, see the m-file getxo.m
      mask Display: dpoly(N,D,'s')
  real : Subsystem  mask(Transfer Function with Initial Outputs){N=[1], D=[to 1], Y0=0, U0=0}
      mask prompts: N "Numerator:"; D "Denominator:"; Y0 "Initial output:"; U0 "Initial input:"
      mask help: Vector expressions for numerator, and denominator. Coefficients are in descending powers of s.
      mask init:
      | [A,B,C,Dd]=tf2ss(N,D);if (isempty(Y0));[m,n]=size(A);X0=zeros(1,m); end; if (isempty(U0));[m,p]=size(B);U0=zeros(1,p);end;X0=getxo(A,B,C,Dd,U0,Y0,0);
      mask Help: Specify the initial output for the transfer function.  An optimization routine attempts to determine the appropriate initial states so that the specified initial output is achieved.  For more details, see the m-file getxo.m
      mask Display: dpoly(N,D,'s')
  Out : Outport  VectorParamsAs1DForOutWhenUnconnected=off
  wires:
  Complex to Real-Imag/1 -> real/1(In1)
  Complex to Real-Imag/2 -> imag/1(In1)
  In/1 -> Complex to Real-Imag/1
  Real-Imag to Complex/1 -> Out/1
  real/1(Out1) -> Real-Imag to Complex/1
  imag/1(Out1) -> Real-Imag to Complex/2

== system ZEH_PV_grid/L11/Load ==
  1 : Constant
  Add : Sum
  Clock : Clock
  Constant : Constant
  Constant1 : Constant  Value=15/24
  Divide : Product  Inputs=*/
  Manual Switch : ManualSwitch
  Mux : Mux  Inputs=2
  P nom : Constant  Value=-nomPower*1e6
  Power consumption : Lookup_n-D  NumberOfTableDimensions=1  BreakpointsForDimension1=[1:timestep/60:24]  BeginIndexSearchUsingPreviousIndexResult=on  Table=datas  InternalRulePriority=Speed  RndMeth=Simplest  InputSameDT=on
  Power factor : Constant  Value=PF^2
  Product : Product
  Product1 : Product
  Scope : Scope
  Second-->Hour : Gain  Gain=1/(60*60)
  Sqrt : Sqrt  SaturateOnIntegerOverflow=on
  Sum : Sum  Inputs=-+
  PQ : Outport  VectorParamsAs1DForOutWhenUnconnected=off
  wires:
  Constant/1 -> Add/2
  1/1 -> Sum/1, Divide/1
  Second-->Hour/1 -> Add/1
  Sum/1 -> Sqrt/1
  Power factor/1 -> Divide/2
  Add/1 -> Power consumption/1
  P nom/1 -> Product/2
  Clock/1 -> Second-->Hour/1
  Sqrt/1 -> Product1/2
  Product/1 -> Product1/1, Mux/1
  Divide/1 -> Sum/2
  Product1/1 -> Mux/2
  Power consumption/1 -> Manual Switch/1
  Manual Switch/1 -> Product/1
  Constant1/1 -> Manual Switch/2
  Mux/1 -> Scope/1, PQ/1

== system ZEH_PV_grid/L2/Avoid division by zero ==
  I : Inport
  Complex to Magnitude-Angle : ComplexToMagnitudeAngle
  Magnitude-Angle to Complex : MagnitudeAngleToComplex
  Saturation1 : Saturate  UpperLimit=inf  LowerLimit=1e-6
  O : Outport  VectorParamsAs1DForOutWhenUnconnected=off
  wires:
  Complex to Magnitude-Angle/2 -> Magnitude-Angle to Complex/2
  Magnitude-Angle to Complex/1 -> O/1
  Complex to Magnitude-Angle/1 -> Saturation1/1
  Saturation1/1 -> Magnitude-Angle to Complex/1
  I/1 -> Complex to Magnitude-Angle/1

== system ZEH_PV_grid/L2/Break Alg. Loop 1 ==
  In : Inport
  Complex to Real-Imag : ComplexToRealImag
  Real-Imag to Complex : RealImagToComplex
  imag : Subsystem  mask(Transfer Function with Initial Outputs){N=[1], D=[to  1], Y0=0, U0=0}
      mask prompts: N "Numerator:"; D "Denominator:"; Y0 "Initial output:"; U0 "Initial input:"
      mask help: Vector expressions for numerator, and denominator. Coefficients are in descending powers of s.
      mask init:
      | [A,B,C,Dd]=tf2ss(N,D);if (isempty(Y0));[m,n]=size(A);X0=zeros(1,m); end; if (isempty(U0));[m,p]=size(B);U0=zeros(1,p);end;X0=getxo(A,B,C,Dd,U0,Y0,0);
      mask Help: Specify the initial output for the transfer function.  An optimization routine attempts to determine the appropriate initial states so that the specified initial output is achieved.  For more details, see the m-file getxo.m
      mask Display: dpoly(N,D,'s')
  real : Subsystem  mask(Transfer Function with Initial Outputs){N=[1], D=[to 1], Y0=0, U0=0}
      mask prompts: N "Numerator:"; D "Denominator:"; Y0 "Initial output:"; U0 "Initial input:"
      mask help: Vector expressions for numerator, and denominator. Coefficients are in descending powers of s.
      mask init:
      | [A,B,C,Dd]=tf2ss(N,D);if (isempty(Y0));[m,n]=size(A);X0=zeros(1,m); end; if (isempty(U0));[m,p]=size(B);U0=zeros(1,p);end;X0=getxo(A,B,C,Dd,U0,Y0,0);
      mask Help: Specify the initial output for the transfer function.  An optimization routine attempts to determine the appropriate initial states so that the specified initial output is achieved.  For more details, see the m-file getxo.m
      mask Display: dpoly(N,D,'s')
  Out : Outport  VectorParamsAs1DForOutWhenUnconnected=off
  wires:
  imag/1(Out1) -> Real-Imag to Complex/2
  real/1(Out1) -> Real-Imag to Complex/1
  Real-Imag to Complex/1 -> Out/1
  In/1 -> Complex to Real-Imag/1
  Complex to Real-Imag/2 -> imag/1(In1)
  Complex to Real-Imag/1 -> real/1(In1)

== system ZEH_PV_grid/L2/Load ==
  1 : Constant
  Add : Sum
  Clock : Clock
  Constant : Constant
  Constant1 : Constant  Value=15/24
  Divide : Product  Inputs=*/
  Manual Switch : ManualSwitch
  Mux : Mux  Inputs=2
  P nom : Constant  Value=-nomPower*1e6
  Power consumption : Lookup_n-D  NumberOfTableDimensions=1  BreakpointsForDimension1=[1:timestep/60:24]  BeginIndexSearchUsingPreviousIndexResult=on  Table=datas  InternalRulePriority=Speed  RndMeth=Simplest  InputSameDT=on
  Power factor : Constant  Value=PF^2
  Product : Product
  Product1 : Product
  Scope : Scope
  Second-->Hour : Gain  Gain=1/(60*60)
  Sqrt : Sqrt  SaturateOnIntegerOverflow=on
  Sum : Sum  Inputs=-+
  PQ : Outport  VectorParamsAs1DForOutWhenUnconnected=off
  wires:
  Mux/1 -> PQ/1, Scope/1
  Constant1/1 -> Manual Switch/2
  Manual Switch/1 -> Product/1
  Power consumption/1 -> Manual Switch/1
  Product1/1 -> Mux/2
  Divide/1 -> Sum/2
  Product/1 -> Mux/1, Product1/1
  Sqrt/1 -> Product1/2
  Clock/1 -> Second-->Hour/1
  P nom/1 -> Product/2
  Add/1 -> Power consumption/1
  Power factor/1 -> Divide/2
  Sum/1 -> Sqrt/1
  Second-->Hour/1 -> Add/1
  1/1 -> Divide/1, Sum/1
  Constant/1 -> Add/2

== system ZEH_PV_grid/L3/Avoid division by zero ==
  I : Inport
  Complex to Magnitude-Angle : ComplexToMagnitudeAngle
  Magnitude-Angle to Complex : MagnitudeAngleToComplex
  Saturation1 : Saturate  UpperLimit=inf  LowerLimit=1e-6
  O : Outport  VectorParamsAs1DForOutWhenUnconnected=off
  wires:
  I/1 -> Complex to Magnitude-Angle/1
  Saturation1/1 -> Magnitude-Angle to Complex/1
  Complex to Magnitude-Angle/1 -> Saturation1/1
  Magnitude-Angle to Complex/1 -> O/1
  Complex to Magnitude-Angle/2 -> Magnitude-Angle to Complex/2

== system ZEH_PV_grid/L3/Break Alg. Loop 1 ==
  In : Inport
  Complex to Real-Imag : ComplexToRealImag
  Real-Imag to Complex : RealImagToComplex
  imag : Subsystem  mask(Transfer Function with Initial Outputs){N=[1], D=[to  1], Y0=0, U0=0}
      mask prompts: N "Numerator:"; D "Denominator:"; Y0 "Initial output:"; U0 "Initial input:"
      mask help: Vector expressions for numerator, and denominator. Coefficients are in descending powers of s.
      mask init:
      | [A,B,C,Dd]=tf2ss(N,D);if (isempty(Y0));[m,n]=size(A);X0=zeros(1,m); end; if (isempty(U0));[m,p]=size(B);U0=zeros(1,p);end;X0=getxo(A,B,C,Dd,U0,Y0,0);
      mask Help: Specify the initial output for the transfer function.  An optimization routine attempts to determine the appropriate initial states so that the specified initial output is achieved.  For more details, see the m-file getxo.m
      mask Display: dpoly(N,D,'s')
  real : Subsystem  mask(Transfer Function with Initial Outputs){N=[1], D=[to 1], Y0=0, U0=0}
      mask prompts: N "Numerator:"; D "Denominator:"; Y0 "Initial output:"; U0 "Initial input:"
      mask help: Vector expressions for numerator, and denominator. Coefficients are in descending powers of s.
      mask init:
      | [A,B,C,Dd]=tf2ss(N,D);if (isempty(Y0));[m,n]=size(A);X0=zeros(1,m); end; if (isempty(U0));[m,p]=size(B);U0=zeros(1,p);end;X0=getxo(A,B,C,Dd,U0,Y0,0);
      mask Help: Specify the initial output for the transfer function.  An optimization routine attempts to determine the appropriate initial states so that the specified initial output is achieved.  For more details, see the m-file getxo.m
      mask Display: dpoly(N,D,'s')
  Out : Outport  VectorParamsAs1DForOutWhenUnconnected=off
  wires:
  Complex to Real-Imag/1 -> real/1(In1)
  Complex to Real-Imag/2 -> imag/1(In1)
  In/1 -> Complex to Real-Imag/1
  Real-Imag to Complex/1 -> Out/1
  real/1(Out1) -> Real-Imag to Complex/1
  imag/1(Out1) -> Real-Imag to Complex/2

== system ZEH_PV_grid/L3/Load ==
  1 : Constant
  Add : Sum
  Clock : Clock
  Constant : Constant
  Constant1 : Constant  Value=15/24
  Divide : Product  Inputs=*/
  Manual Switch : ManualSwitch
  Mux : Mux  Inputs=2
  P nom : Constant  Value=-nomPower*1e6
  Power consumption : Lookup_n-D  NumberOfTableDimensions=1  BreakpointsForDimension1=[1:timestep/60:24]  BeginIndexSearchUsingPreviousIndexResult=on  Table=datas  InternalRulePriority=Speed  RndMeth=Simplest  InputSameDT=on
  Power factor : Constant  Value=PF^2
  Product : Product
  Product1 : Product
  Scope : Scope
  Second-->Hour : Gain  Gain=1/(60*60)
  Sqrt : Sqrt  SaturateOnIntegerOverflow=on
  Sum : Sum  Inputs=-+
  PQ : Outport  VectorParamsAs1DForOutWhenUnconnected=off
  wires:
  Constant/1 -> Add/2
  1/1 -> Sum/1, Divide/1
  Second-->Hour/1 -> Add/1
  Sum/1 -> Sqrt/1
  Power factor/1 -> Divide/2
  Add/1 -> Power consumption/1
  P nom/1 -> Product/2
  Clock/1 -> Second-->Hour/1
  Sqrt/1 -> Product1/2
  Product/1 -> Product1/1, Mux/1
  Divide/1 -> Sum/2
  Product1/1 -> Mux/2
  Power consumption/1 -> Manual Switch/1
  Manual Switch/1 -> Product/1
  Constant1/1 -> Manual Switch/2
  Mux/1 -> Scope/1, PQ/1

== system ZEH_PV_grid/L4/Avoid division by zero ==
  I : Inport
  Complex to Magnitude-Angle : ComplexToMagnitudeAngle
  Magnitude-Angle to Complex : MagnitudeAngleToComplex
  Saturation1 : Saturate  UpperLimit=inf  LowerLimit=1e-6
  O : Outport  VectorParamsAs1DForOutWhenUnconnected=off
  wires:
  Complex to Magnitude-Angle/2 -> Magnitude-Angle to Complex/2
  Magnitude-Angle to Complex/1 -> O/1
  Complex to Magnitude-Angle/1 -> Saturation1/1
  Saturation1/1 -> Magnitude-Angle to Complex/1
  I/1 -> Complex to Magnitude-Angle/1

== system ZEH_PV_grid/L4/Break Alg. Loop 1 ==
  In : Inport
  Complex to Real-Imag : ComplexToRealImag
  Real-Imag to Complex : RealImagToComplex
  imag : Subsystem  mask(Transfer Function with Initial Outputs){N=[1], D=[to  1], Y0=0, U0=0}
      mask prompts: N "Numerator:"; D "Denominator:"; Y0 "Initial output:"; U0 "Initial input:"
      mask help: Vector expressions for numerator, and denominator. Coefficients are in descending powers of s.
      mask init:
      | [A,B,C,Dd]=tf2ss(N,D);if (isempty(Y0));[m,n]=size(A);X0=zeros(1,m); end; if (isempty(U0));[m,p]=size(B);U0=zeros(1,p);end;X0=getxo(A,B,C,Dd,U0,Y0,0);
      mask Help: Specify the initial output for the transfer function.  An optimization routine attempts to determine the appropriate initial states so that the specified initial output is achieved.  For more details, see the m-file getxo.m
      mask Display: dpoly(N,D,'s')
  real : Subsystem  mask(Transfer Function with Initial Outputs){N=[1], D=[to 1], Y0=0, U0=0}
      mask prompts: N "Numerator:"; D "Denominator:"; Y0 "Initial output:"; U0 "Initial input:"
      mask help: Vector expressions for numerator, and denominator. Coefficients are in descending powers of s.
      mask init:
      | [A,B,C,Dd]=tf2ss(N,D);if (isempty(Y0));[m,n]=size(A);X0=zeros(1,m); end; if (isempty(U0));[m,p]=size(B);U0=zeros(1,p);end;X0=getxo(A,B,C,Dd,U0,Y0,0);
      mask Help: Specify the initial output for the transfer function.  An optimization routine attempts to determine the appropriate initial states so that the specified initial output is achieved.  For more details, see the m-file getxo.m
      mask Display: dpoly(N,D,'s')
  Out : Outport  VectorParamsAs1DForOutWhenUnconnected=off
  wires:
  imag/1(Out1) -> Real-Imag to Complex/2
  real/1(Out1) -> Real-Imag to Complex/1
  Real-Imag to Complex/1 -> Out/1
  In/1 -> Complex to Real-Imag/1
  Complex to Real-Imag/2 -> imag/1(In1)
  Complex to Real-Imag/1 -> real/1(In1)

== system ZEH_PV_grid/L4/Load ==
  1 : Constant
  Add : Sum
  Clock : Clock
  Constant : Constant
  Constant1 : Constant  Value=15/24
  Divide : Product  Inputs=*/
  Manual Switch : ManualSwitch
  Mux : Mux  Inputs=2
  P nom : Constant  Value=-nomPower*1e6
  Power consumption : Lookup_n-D  NumberOfTableDimensions=1  BreakpointsForDimension1=[1:timestep/60:24]  BeginIndexSearchUsingPreviousIndexResult=on  Table=datas  InternalRulePriority=Speed  RndMeth=Simplest  InputSameDT=on
  Power factor : Constant  Value=PF^2
  Product : Product
  Product1 : Product
  Scope : Scope
  Second-->Hour : Gain  Gain=1/(60*60)
  Sqrt : Sqrt  SaturateOnIntegerOverflow=on
  Sum : Sum  Inputs=-+
  PQ : Outport  VectorParamsAs1DForOutWhenUnconnected=off
  wires:
  Mux/1 -> PQ/1, Scope/1
  Constant1/1 -> Manual Switch/2
  Manual Switch/1 -> Product/1
  Power consumption/1 -> Manual Switch/1
  Product1/1 -> Mux/2
  Divide/1 -> Sum/2
  Product/1 -> Mux/1, Product1/1
  Sqrt/1 -> Product1/2
  Clock/1 -> Second-->Hour/1
  P nom/1 -> Product/2
  Add/1 -> Power consumption/1
  Power factor/1 -> Divide/2
  Sum/1 -> Sqrt/1
  Second-->Hour/1 -> Add/1
  1/1 -> Divide/1, Sum/1
  Constant/1 -> Add/2
